simulink model "bicycle_model"  (R2025a)
settings: Solver=VariableStepAuto  StartTime=0.0  StopTime=40  RelTol=1e-3
undefined symbols (not defined in the file): k, Kd, Ki, Kp, L, max_delta
libraries: simulink x1
settings Model: Creator=王以乐  LastModifiedBy=王以乐

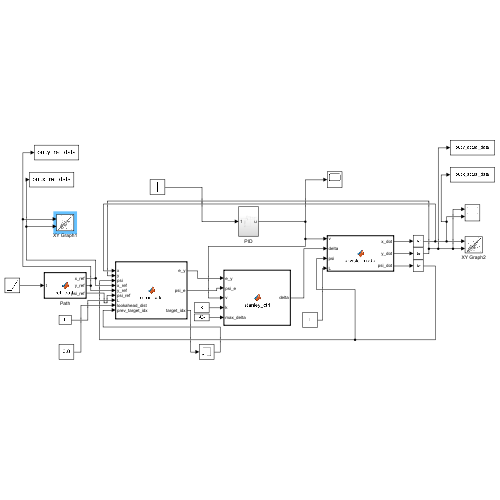
[thumbnail: Simulink's stored preview of the top-level diagram]
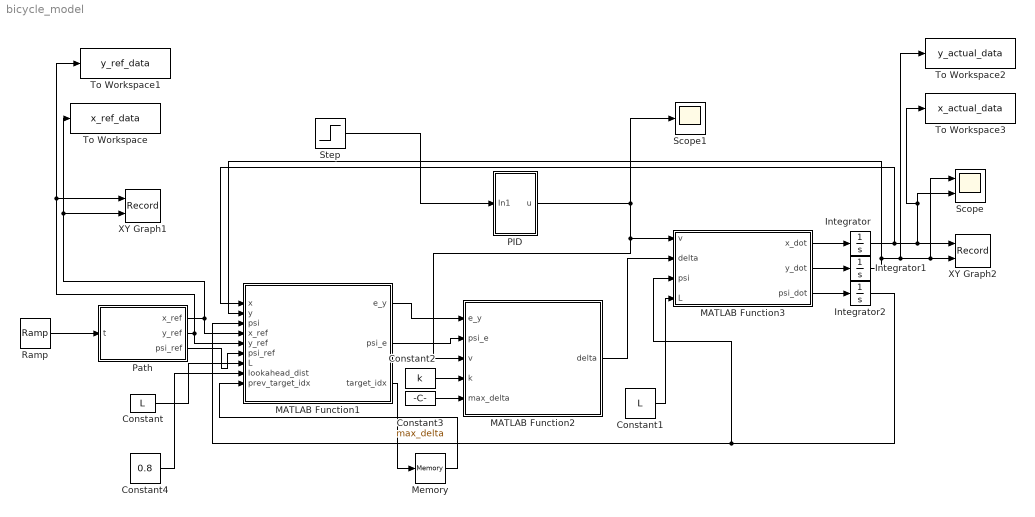
== system bicycle_model ==
  Constant : Constant  Value=L
  Constant1 : Constant  Value=L
  Constant2 : Constant  Value=k
  Constant3 : Constant  Value=max_delta
  Constant4 : Constant  Value=0.8
  Integrator : Integrator
  Integrator1 : Integrator
  Integrator2 : Integrator
  MATLAB Function1 : MATLAB Function  TreatAsAtomicUnit=on
  MATLAB Function2 : MATLAB Function  TreatAsAtomicUnit=on
  MATLAB Function3 : MATLAB Function  TreatAsAtomicUnit=on
  Memory : Memory
  PID : Subsystem
  Path : MATLAB Function  TreatAsAtomicUnit=on
  Ramp : simulink/Sources/Ramp  slope=1  start=0  InitialOutput=0
  Scope : Scope  NumInputPorts=2
      settings: ActiveDisplayYMinimum=-138.814106213743  ActiveDisplayYMaximum=118.52553319491165
  Scope1 : Scope
      settings: ActiveDisplayYMinimum=-7.0416644111394291  ActiveDisplayYMaximum=6.7566190786361542
  Step : Step  Time=0  SampleTime=0
  To Workspace : ToWorkspace  VariableName=x_ref_data  SampleTime=-1
  To Workspace1 : ToWorkspace  VariableName=y_ref_data  SampleTime=-1
  To Workspace2 : ToWorkspace  VariableName=y_actual_data  SampleTime=-1
  To Workspace3 : ToWorkspace  VariableName=x_actual_data  SampleTime=-1
  XY Graph1 : Record  NumPorts=2.0  FileSettingsInternal="{\"entries\":[{\"content\":{\"excelSettings\":{\"content\":{},\"type\":\"Streamout.ExcelSettings\"},\"parquetSettings\":{\"content\":{},\"type\":\"Streamout.ParquetSettings\"}},\"type\":\"Streamout.FileSettingStorage\",\"uuid\":\"\"}],\"packageUris\":[\"http:\\/\\/schema.mathworks.com\\/mf0\\/streamout_blocks\\/R2020a\"],\"version\":\"1.0\"}"  FrameSettings=[0, 0]  Layout=[1 1]  SignalsInternal="{\"entries\":[{\"content\":{\"signals\":[{\"content\":{\"blockPath\":[],\"dimensions\":[1],\"domain\":\"\",\"lineColor\":\"#a2142f\",\"plots\":[ 1 ],\"port\":1,\"sid\":[\"\"],\"signalID\":1,\"signalName\":\"Path:2\"},\"type\":\"RecordBlkView.Signal\",\"uuid\":\"\"},{\"content\":{\"blockPath\":[],\"dimensions\":[1],\"domain\":\"\",\"lineColor\":\"#139fff\",\"plots\":[ 1 ],\"port\":2,\"sid\":[\"\"],\"signalID\":2,\"signalName\":\"Path:1\"},\"type\":\"RecordBlkView.Signal\",\"uuid\":\"\"}]},\"type\":\"RecordBlkView.InputSignals\",\"uuid\":\"\"}],\"packageUris\":[\"http:\\/\\/schema.mathworks.com\\/mf0\\/streamout_blocks\\/R2020a\"],\"version\":\"1.0\"}"  VisualizationBindings="{\"xyplotplugin\":{\"info\":[{\"series\":[{\"bindingParametersList\":[{\"parameter\":\"X-Axis\",\"signalID\":2,\"signalName\":\"Path:1\"},{\"parameter\":\"Y-Axis\",\"signalID\":1,\"signalName\":\"Path:2\"}],\"seriesID\":0}],\"subplotID\":1}]}}"  CompatibilityTag=XY
  XY Graph2 : Record  NumPorts=2.0  FileSettingsInternal="{\"entries\":[{\"content\":{\"excelSettings\":{\"content\":{},\"type\":\"Streamout.ExcelSettings\"},\"parquetSettings\":{\"content\":{},\"type\":\"Streamout.ParquetSettings\"}},\"type\":\"Streamout.FileSettingStorage\",\"uuid\":\"\"}],\"packageUris\":[\"http:\\/\\/schema.mathworks.com\\/mf0\\/streamout_blocks\\/R2020a\"],\"version\":\"1.0\"}"  FrameSettings=[0, 0]  Layout=[1 1]  SignalsInternal="{\"entries\":[{\"content\":{\"signals\":[{\"content\":{\"blockPath\":[],\"dimensions\":[1],\"domain\":\"\",\"lineColor\":\"#a2142f\",\"plots\":[ 1 ],\"port\":1,\"sid\":[\"\"],\"signalID\":1,\"signalName\":\"Integrator\"},\"type\":\"RecordBlkView.Signal\",\"uuid\":\"\"},{\"content\":{\"blockPath\":[],\"dimensions\":[1],\"domain\":\"\",\"lineColor\":\"#139fff\",\"plots\":[ 1 ],\"port\":2,\"sid\":[\"\"],\"signalID\":2,\"signalName\":\"Integrator1\"},\"type\":\"RecordBlkView.Signal\",\"uuid\":\"\"}]},\"type\":\"RecordBlkView.InputSignals\",\"uuid\":\"\"}],\"packageUris\":[\"http:\\/\\/schema.mathworks.com\\/mf0\\/streamout_blocks\\/R2020a\"],\"version\":\"1.0\"}"  VisualizationBindings="{\"xyplotplugin\":{\"info\":[{\"series\":[{\"bindingParametersList\":[{\"parameter\":\"X-Axis\",\"signalID\":1,\"signalName\":\"Integrator\"},{\"parameter\":\"Y-Axis\",\"signalID\":2,\"signalName\":\"Integrator1\"}],\"seriesID\":0}],\"subplotID\":1}]}}"  CompatibilityTag=XY
  wires:
  Step/1 -> PID/1(In1)
  PID/1(u) -> MATLAB Function2/3(v), MATLAB Function3/1(v), Scope1/1
  Constant1/1 -> MATLAB Function3/4(L)
  Path/1(x_ref) -> To Workspace/1, XY Graph1/2, MATLAB Function1/4(x_ref)
  Path/2(y_ref) -> To Workspace1/1, XY Graph1/1, MATLAB Function1/5(y_ref)
  Path/3(psi_ref) -> MATLAB Function1/6(psi_ref)
  Constant/1 -> MATLAB Function1/7(L)
  MATLAB Function1/1(e_y) -> MATLAB Function2/1(e_y)
  MATLAB Function1/2(psi_e) -> MATLAB Function2/2(psi_e)
  MATLAB Function2/1(delta) -> MATLAB Function3/2(delta)
  MATLAB Function3/1(x_dot) -> Integrator/1
  MATLAB Function3/2(y_dot) -> Integrator1/1
  MATLAB Function3/3(psi_dot) -> Integrator2/1
  Integrator/1 -> MATLAB Function1/1(x), To Workspace3/1, Scope/2, XY Graph2/1
  Integrator1/1 -> Scope/1, XY Graph2/2, To Workspace2/1, MATLAB Function1/2(y)
  Integrator2/1 -> MATLAB Function3/3(psi), MATLAB Function1/3(psi)
  Constant2/1 -> MATLAB Function2/4(k)
  Constant3/1 -> MATLAB Function2/5(max_delta)
  Ramp/1 -> Path/1(t)
  MATLAB Function1/3(target_idx) -> Memory/1
  Memory/1 -> MATLAB Function1/9(prev_target_idx)
  Constant4/1 -> MATLAB Function1/8(lookahead_dist)

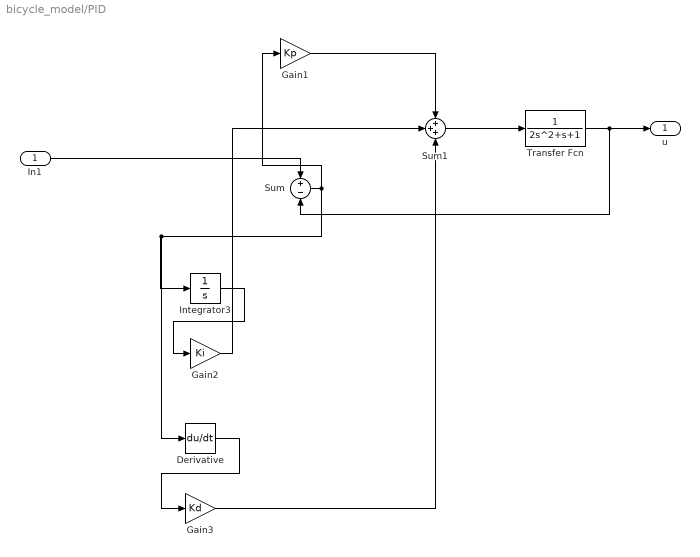
== system bicycle_model/PID ==
  In1 : Inport
  Derivative : Derivative
  Gain1 : Gain  Gain=Kp
  Gain2 : Gain  Gain=Ki
  Gain3 : Gain  Gain=Kd
  Integrator3 : Integrator
  Sum : Sum  Inputs=+-
  Sum1 : Sum  Inputs=+++
  Transfer Fcn : TransferFcn  Denominator=[2 1 1]
  u : Outport
  wires:
  Derivative/1 -> Gain3/1
  Gain1/1 -> Sum1/1
  Sum/1 -> Derivative/1, Integrator3/1, Gain1/1
  Gain3/1 -> Sum1/3
  Sum1/1 -> Transfer Fcn/1
  Integrator3/1 -> Gain2/1
  Gain2/1 -> Sum1/2
  Transfer Fcn/1 -> u/1, Sum/2
  In1/1 -> Sum/1

== matlab function bicycle_model/MATLAB Function1 ==
  data: x input; e_y output; psi_e output; y input; psi input; x_ref input; y_ref input; psi_ref input; L input; lookahead_dist input; prev_target_idx input; target_idx output
function [e_y, psi_e, target_idx] = error_calc(x, y, psi, x_ref, y_ref, psi_ref, L, lookahead_dist, prev_target_idx)
    % 输入参数:
    % lookahead_dist: 预瞄距离(米)，推荐值: 车辆速度*0.8
    % prev_target_idx: 上一时刻的目标点索引(用于连续性约束)
    
    % 1. 计算前轮位置
    x_front = x + L * cos(psi);
    y_front = y + L * sin(psi);
    
    % 2. 生成预瞄点(沿车辆航向方向延伸)
    x_lookahead = x_front + lookahead_dist * cos(psi);
    y_lookahead = y_front + lookahead_dist * sin(psi);
    
    % 3. 计算预瞄点到路径各点的距离
    distances = sqrt((x_ref - x_lookahead).^2 + (y_ref - y_lookahead).^2);
    
    % 4. 添加方向约束(只考虑车辆前方的路径点)
    path_directions = [x_ref - x_front; y_ref - y_front];  % 路径点相对于前轮的方向向量
    vehicle_direction = [cos(psi); sin(psi)];  % 车辆前进方向单位向量
    
    % 计算点积(点积>0表示在车辆前进方向上)
    dot_products = path_directions(1,:) .* vehicle_direction(1) + path_directions(2,:) .* vehicle_direction(2);
    forward_mask = dot_products > 0;
    
    % 排除非前进方向的点
    filtered_distances = distances;
    filtered_distances(~forward_mask) = inf;
    
    % 5. 添加历史连续性约束(优先选择上一目标点附近的点)
    if nargin >= 9 && ~isempty(prev_target_idx)
        % 设置搜索窗口(通常为上一目标点前后各10个点)
        window_size = 10;
        window_start = max(1, prev_target_idx - window_size);
        window_end = min(length(x_ref), prev_target_idx + window_size);
        
        % 创建窗口掩码
        window_mask = false(1, length(x_ref));
        window_mask(window_start:window_end) = true;
        
        % 仅在窗口内搜索
        filtered_distances(~window_mask) = inf;
    end
    
    % 6. 选择最终目标点
    [~, target_idx] = min(filtered_distances);
    
    % 7. 获取目标点的参考路径信息
    x_ref_target = x_ref(target_idx);
    y_ref_target = y_ref(target_idx);
    psi_ref_target = psi_ref(target_idx);
    
    % 8. 计算横向误差(前轮位置到目标点的法向投影)
    t_vec = [cos(psi_ref_target); sin(psi_ref_target)];  % 参考路径切线向量
    n_vec = [-sin(psi_ref_target); cos(psi_ref_target)]; % 参考路径法线向量(指向路径左侧为正)
    
    % 计算前轮到目标点的向量
    target_vec = [x_front - x_ref_target; y_front - y_ref_target];
    
    % 计算横向误差(向量在法线方向上的投影)
    e_y = dot(target_vec, n_vec);  % 右侧为正，左侧为负
    
    % 9. 计算航向误差(归一化到[-pi, pi])
    psi_e = psi_ref_target - psi;
    
    % 确保误差在[-pi, pi]范围内
    if psi_e > pi
        psi_e = psi_e - 2*pi;
    elseif psi_e < -pi
        psi_e = psi_e + 2*pi;
    end
end

== matlab function bicycle_model/Path ==
  data: t input; x_ref output; y_ref output; psi_ref output
function [x_ref, y_ref, psi_ref] = ref_path(t)
    R = 10;        % 路径半径（m）
    omega = 0.1;   % 角速度（rad/s）
    s = omega * t; % 弧长参数
    
    % 调整初始相位，使t=0时从(0,0)开始
    x_ref = R * sin(s);  % 初始点(0,0)
    y_ref = -R * (1 - cos(s));        % 初始点(0,0) 
    psi_ref = atan2(y_ref, x_ref);  % 路径切线方向
end

== matlab function bicycle_model/MATLAB Function2 ==
  data: e_y input; delta output; psi_e input; v input; k input; max_delta input
function delta = stanley_ctrl(e_y, psi_e, v, k, max_delta)
    % Stanley 算法核心公式
    delta = -psi_e - atan2(k * e_y, v);
    
    % 限制前轮偏角范围
    delta = max(min(delta, max_delta), -max_delta);
end

== matlab function bicycle_model/MATLAB Function3 ==
  data: v input; delta input; psi input; x_dot output; L input; y_dot output; psi_dot output
function [x_dot, y_dot, psi_dot] = bicycle_model(v, delta, psi, L)
    % 仅计算导数，不更新状态
    x_dot = v * cos(psi);
    y_dot = v * sin(psi);
    psi_dot = (v/L) * tan(delta);
end
